simulink model "car_model_spl_heur3"  (R2020b)
settings: Solver=FixedStepAuto  StartTime=0.0  StopTime=45  FixedStep=0.05  RelTol=1e-3
undefined symbols (not defined in the file or in its folder): theta0, x0, y0
settings Model: Creator=Lexa  LastModifiedBy=msw
settings SolverCC: AlgebraicLoopSolver=LineSearch
settings DebuggingCC: UnderSpecifiedDimensionMsg=error
settings SFSimCC: CustomCodeUndefinedFunction=UseInterfaceOnly

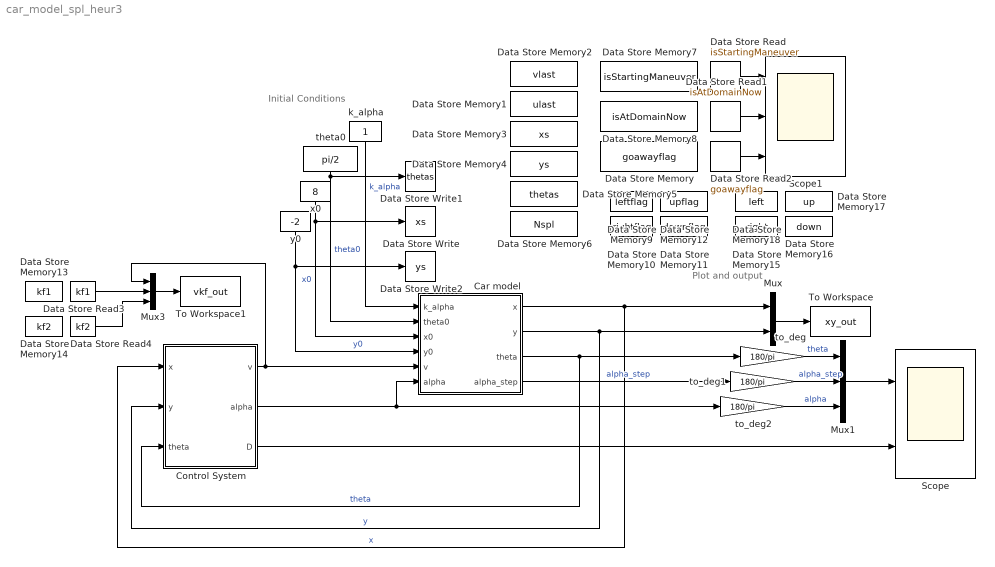
== system car_model_spl_heur3 ==
  note: Plot and output
  note: Initial Conditions
  Car model : Subsystem
      mask Display: image('car_model.png');
  Control System : Subsystem  StopFcn=close all
  Data Store Memory : DataStoreMemory  DataStoreName=goawayflag  ReadBeforeWriteMsg=warning  WriteAfterWriteMsg=warning  WriteAfterReadMsg=warning  ShowAdditionalParam=off  OutDataTypeStr=double
  Data Store Memory1 : DataStoreMemory  DataStoreName=ulast  ReadBeforeWriteMsg=warning  WriteAfterWriteMsg=warning  WriteAfterReadMsg=warning  ShowAdditionalParam=off  OutDataTypeStr=double
  Data Store Memory10 : DataStoreMemory  DataStoreName=rightflag  ReadBeforeWriteMsg=warning  WriteAfterWriteMsg=warning  WriteAfterReadMsg=warning  ShowAdditionalParam=off  OutDataTypeStr=double
  Data Store Memory11 : DataStoreMemory  DataStoreName=downflag  ReadBeforeWriteMsg=warning  WriteAfterWriteMsg=warning  WriteAfterReadMsg=warning  ShowAdditionalParam=off  OutDataTypeStr=double
  Data Store Memory12 : DataStoreMemory  DataStoreName=upflag  ReadBeforeWriteMsg=warning  WriteAfterWriteMsg=warning  WriteAfterReadMsg=warning  ShowAdditionalParam=off  OutDataTypeStr=double
  Data Store Memory13 : DataStoreMemory  DataStoreName=kf1  ReadBeforeWriteMsg=warning  WriteAfterWriteMsg=warning  WriteAfterReadMsg=warning  ShowAdditionalParam=off  OutDataTypeStr=double
  Data Store Memory14 : DataStoreMemory  DataStoreName=kf2  ReadBeforeWriteMsg=warning  WriteAfterWriteMsg=warning  WriteAfterReadMsg=warning  ShowAdditionalParam=off  OutDataTypeStr=double
  Data Store Memory15 : DataStoreMemory  DataStoreName=right  ReadBeforeWriteMsg=warning  WriteAfterWriteMsg=warning  WriteAfterReadMsg=warning  ShowAdditionalParam=off  OutDataTypeStr=double
  Data Store Memory16 : DataStoreMemory  DataStoreName=down  ReadBeforeWriteMsg=warning  WriteAfterWriteMsg=warning  WriteAfterReadMsg=warning  ShowAdditionalParam=off  OutDataTypeStr=double
  Data Store Memory17 : DataStoreMemory  DataStoreName=up  ReadBeforeWriteMsg=warning  WriteAfterWriteMsg=warning  WriteAfterReadMsg=warning  ShowAdditionalParam=off  OutDataTypeStr=double
  Data Store Memory18 : DataStoreMemory  DataStoreName=left  ReadBeforeWriteMsg=warning  WriteAfterWriteMsg=warning  WriteAfterReadMsg=warning  ShowAdditionalParam=off  OutDataTypeStr=double
  Data Store Memory2 : DataStoreMemory  DataStoreName=vlast  ReadBeforeWriteMsg=warning  WriteAfterWriteMsg=warning  WriteAfterReadMsg=warning  ShowAdditionalParam=off  OutDataTypeStr=double
  Data Store Memory3 : DataStoreMemory  DataStoreName=xs  ReadBeforeWriteMsg=warning  WriteAfterWriteMsg=warning  WriteAfterReadMsg=warning  ShowAdditionalParam=off  OutDataTypeStr=double
  Data Store Memory4 : DataStoreMemory  DataStoreName=ys  ReadBeforeWriteMsg=warning  WriteAfterWriteMsg=warning  WriteAfterReadMsg=warning  ShowAdditionalParam=off  OutDataTypeStr=double
  Data Store Memory5 : DataStoreMemory  DataStoreName=thetas  ReadBeforeWriteMsg=warning  WriteAfterWriteMsg=warning  WriteAfterReadMsg=warning  ShowAdditionalParam=off  OutDataTypeStr=double
  Data Store Memory6 : DataStoreMemory  DataStoreName=Nspl  ReadBeforeWriteMsg=warning  WriteAfterWriteMsg=warning  WriteAfterReadMsg=warning  ShowAdditionalParam=off  OutDataTypeStr=double
  Data Store Memory7 : DataStoreMemory  DataStoreName=isStartingManeuver  ReadBeforeWriteMsg=warning  WriteAfterWriteMsg=warning  WriteAfterReadMsg=warning  ShowAdditionalParam=off  OutDataTypeStr=double
  Data Store Memory8 : DataStoreMemory  DataStoreName=isAtDomainNow  ReadBeforeWriteMsg=warning  WriteAfterWriteMsg=warning  WriteAfterReadMsg=warning  ShowAdditionalParam=off  OutDataTypeStr=boolean
  Data Store Memory9 : DataStoreMemory  DataStoreName=leftflag  ReadBeforeWriteMsg=warning  WriteAfterWriteMsg=warning  WriteAfterReadMsg=warning  ShowAdditionalParam=off  OutDataTypeStr=double
  Data Store Read : DataStoreRead  DataStoreName=isStartingManeuver
  Data Store Read1 : DataStoreRead  DataStoreName=isAtDomainNow
  Data Store Read2 : DataStoreRead  DataStoreName=goawayflag
  Data Store Read3 : DataStoreRead  DataStoreName=kf1
  Data Store Read4 : DataStoreRead  DataStoreName=kf2
  Data Store Write : DataStoreWrite  DataStoreName=xs
  Data Store Write1 : DataStoreWrite  DataStoreName=thetas
  Data Store Write2 : DataStoreWrite  DataStoreName=ys
  Mux : Mux  Inputs=2
  Mux1 : Mux  Inputs=3
  Mux3 : Mux  Inputs=3
  Scope : Scope  NumInputPorts=2
  Scope1 : Scope  NumInputPorts=3
  To Workspace : ToWorkspace  VariableName=xy_out  SaveFormat=Timeseries  SampleTime=-1
  To Workspace1 : ToWorkspace  VariableName=vkf_out  SaveFormat=Timeseries  SampleTime=-1
  k_alpha : Constant  VectorParams1D=off
  theta0 : Constant  Value=pi/2  VectorParams1D=off
  to_deg : Gain  Gain=180/pi
  to_deg1 : Gain  Gain=180/pi
  to_deg2 : Gain  Gain=180/pi
  x0 : Constant  Value=8
  y0 : Constant  Value=-2
  wires:
  Mux/1 -> To Workspace/1
  Car model/1(x) -> Control System/1(x), Mux/1  "x"
  Car model/2(y) -> Control System/2(y), Mux/2  "y"
  theta0/1 -> Data Store Write1/1, Car model/2(theta0)  "theta0"
  x0/1 -> Data Store Write/1, Car model/3(x0)  "x0"
  y0/1 -> Data Store Write2/1, Car model/4(y0)  "y0"
  to_deg/1 -> Mux1/1  "theta"
  Car model/4(alpha_step) -> to_deg1/1  "alpha_step"
  to_deg1/1 -> Mux1/2  "alpha_step"
  to_deg2/1 -> Mux1/3  "alpha"
  Mux1/1 -> Scope/1
  Car model/3(theta) -> Control System/3(theta), to_deg/1  "theta"
  Control System/2(alpha) -> Car model/6(alpha), to_deg2/1
  Control System/3(D) -> Scope/2
  Control System/1(v) -> Car model/5(v), Mux3/1
  Data Store Read/1 -> Scope1/1
  Data Store Read1/1 -> Scope1/2
  Data Store Read2/1 -> Scope1/3
  Data Store Read3/1 -> Mux3/2
  Mux3/1 -> To Workspace1/1
  Data Store Read4/1 -> Mux3/3
  k_alpha/1 -> Car model/1(k_alpha)  "k_alpha"

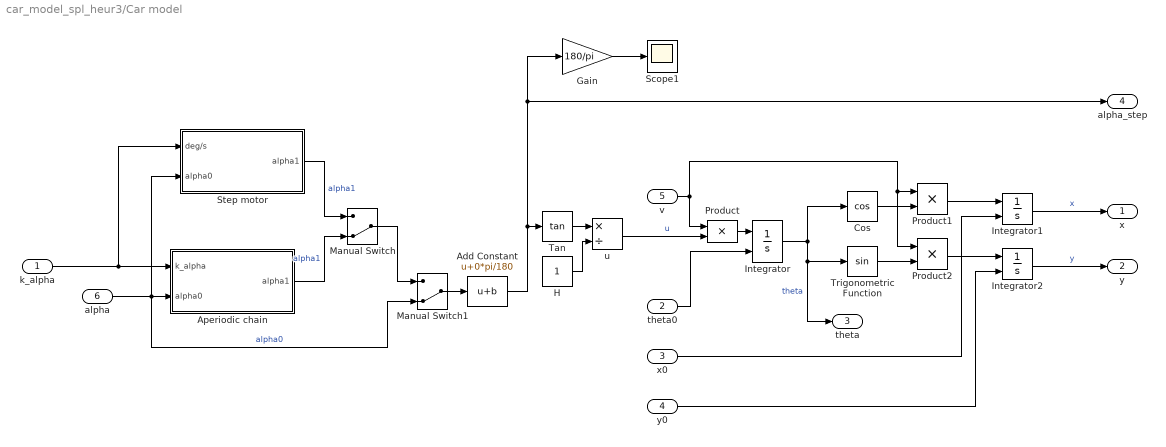
== system car_model_spl_heur3/Car model ==
  k_alpha : Inport
  theta0 : Inport  Port=2
  x0 : Inport  Port=3
  y0 : Inport  Port=4
  v : Inport  Port=5
  alpha : Inport  Port=6
  Add Constant : Bias  Bias=0*pi/180
  Aperiodic chain : Subsystem
  Cos : Trigonometry  Operator=cos
  Gain : Gain  Gain=180/pi
  H : Constant  VectorParams1D=off
  Integrator : Integrator  InitialConditionSource=external  InitialCondition=theta0  WrapState=on
  Integrator1 : Integrator  InitialConditionSource=external  InitialCondition=x0
  Integrator2 : Integrator  InitialConditionSource=external  InitialCondition=y0
  Manual Switch : ManualSwitch  CurrentSetting=0
  Manual Switch1 : ManualSwitch  CurrentSetting=0
  Product : Product
  Product1 : Product
  Product2 : Product
  Scope1 : Scope
  Step motor : Subsystem
  Tan : Trigonometry  Operator=tan
  Trigonometric Function : Trigonometry
  u : Product  Inputs=*/
  x : Outport  VectorParamsAs1DForOutWhenUnconnected=off
  y : Outport  Port=2  VectorParamsAs1DForOutWhenUnconnected=off
  theta : Outport  Port=3  VectorParamsAs1DForOutWhenUnconnected=off
  alpha_step : Outport  Port=4  VectorParamsAs1DForOutWhenUnconnected=off
  wires:
  x0/1 -> Integrator1/2
  Product/1 -> Integrator/1
  Trigonometric Function/1 -> Product2/2
  v/1 -> Product2/1, Product1/1, Product/1
  Integrator/1 -> theta/1, Trigonometric Function/1, Cos/1  "theta"
  Integrator2/1 -> y/1  "y"
  y0/1 -> Integrator2/2
  Integrator1/1 -> x/1  "x"
  Cos/1 -> Product1/2
  Product1/1 -> Integrator1/1
  Product2/1 -> Integrator2/1
  theta0/1 -> Integrator/2
  H/1 -> u/2
  Tan/1 -> u/1
  u/1 -> Product/2  "u"
  alpha/1 -> Manual Switch1/2, Aperiodic chain/2(alpha0), Step motor/2(alpha0)  "alpha0"
  Manual Switch1/1 -> Add Constant/1
  Gain/1 -> Scope1/1
  k_alpha/1 -> Aperiodic chain/1(k_alpha), Step motor/1(deg/s)
  Step motor/1(alpha1) -> Manual Switch/1  "alpha1"
  Aperiodic chain/1(alpha1) -> Manual Switch/2  "alpha1"
  Manual Switch/1 -> Manual Switch1/1
  Add Constant/1 -> Gain/1, alpha_step/1, Tan/1

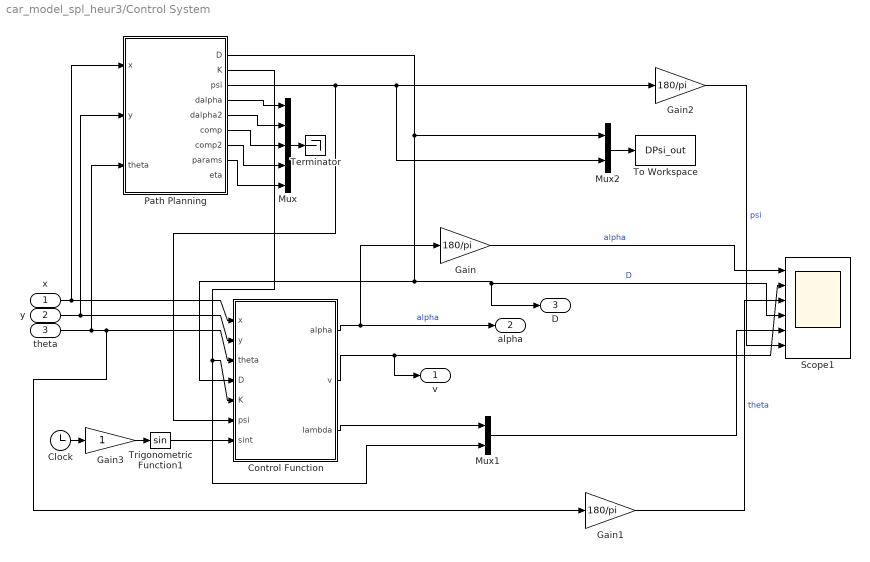
== system car_model_spl_heur3/Control System ==
  x : Inport
  y : Inport  Port=2
  theta : Inport  Port=3
  Clock : Clock
  Control Function : MATLAB Function  TreatAsAtomicUnit=on
  Gain : Gain  Gain=180/pi
  Gain1 : Gain  Gain=180/pi
  Gain2 : Gain  Gain=180/pi
  Gain3 : Gain
  Mux : Mux  Inputs=5
  Mux1 : Mux  Inputs=2
  Mux2 : Mux  Inputs=2
  Path Planning : MATLAB Function  TreatAsAtomicUnit=on
  Scope1 : Scope  NumInputPorts=6
  Terminator : Terminator
  To Workspace : ToWorkspace  VariableName=DPsi_out  SaveFormat=Timeseries  SampleTime=-1
  Trigonometric Function1 : Trigonometry
  v : Outport  VectorParamsAs1DForOutWhenUnconnected=off
  alpha : Outport  Port=2  VectorParamsAs1DForOutWhenUnconnected=off
  D : Outport  Port=3  VectorParamsAs1DForOutWhenUnconnected=off
  wires:
  theta/1 -> Gain1/1, Control Function/3(theta), Path Planning/3(theta)
  Path Planning/1(D) -> Control Function/4(D), Scope1/4, D/1, Mux2/1  "D"
  Control Function/1(alpha) -> alpha/1, Gain/1  "alpha"
  y/1 -> Control Function/2(y), Path Planning/2(y)
  x/1 -> Path Planning/1(x), Control Function/1(x)
  Gain/1 -> Scope1/1  "alpha"
  Path Planning/2(K) -> Mux1/2, Control Function/5(K)
  Path Planning/4(dalpha) -> Mux/1
  Path Planning/5(dalpha2) -> Mux/2
  Path Planning/6(comp) -> Mux/3
  Path Planning/7(comp2) -> Mux/4
  Path Planning/8(params) -> Mux/5
  Gain1/1 -> Scope1/3  "theta"
  Gain2/1 -> Scope1/6  "psi"
  Control Function/3(lambda) -> Mux1/1
  Mux1/1 -> Scope1/5
  Mux2/1 -> To Workspace/1
  Control Function/2(v) -> v/1, Scope1/2
  Mux/1 -> Terminator/1
  Path Planning/3(psi) -> Gain2/1, Mux2/2, Control Function/6(psi)
  Clock/1 -> Gain3/1
  Gain3/1 -> Trigonometric Function1/1
  Trigonometric Function1/1 -> Control Function/7(sint)

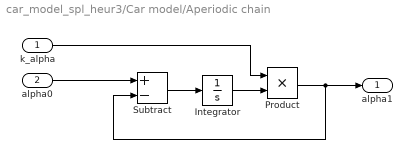
== system car_model_spl_heur3/Car model/Aperiodic chain ==
  k_alpha : Inport
  alpha0 : Inport  Port=2
  Integrator : Integrator
  Product : Product
  Subtract : Sum  Inputs=+-
  alpha1 : Outport  VectorParamsAs1DForOutWhenUnconnected=off
  wires:
  alpha0/1 -> Subtract/1
  Subtract/1 -> Integrator/1
  Integrator/1 -> Product/2
  Product/1 -> Subtract/2, alpha1/1
  k_alpha/1 -> Product/1

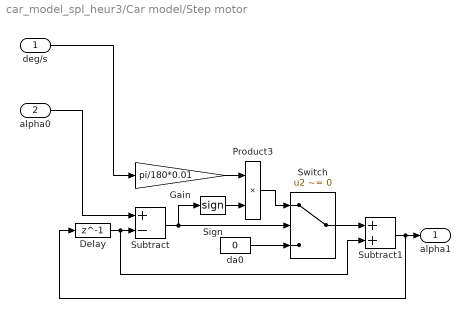
== system car_model_spl_heur3/Car model/Step motor ==
  deg/s : Inport
  alpha0 : Inport  Port=2
  Delay : Delay  DelayLength=1  InitialCondition=0
  Gain : Gain  Gain=pi/180*0.01
  Product3 : Product
  Sign : Signum
  Subtract : Sum  Inputs=+-
  Subtract1 : Sum
  Switch : Switch  Criteria=u2 ~= 0
  da0 : Constant  Value=0  VectorParams1D=off
  alpha1 : Outport  VectorParamsAs1DForOutWhenUnconnected=off
  wires:
  Delay/1 -> Subtract1/2, Subtract/2
  da0/1 -> Switch/3
  deg/s/1 -> Gain/1
  Product3/1 -> Switch/1
  alpha0/1 -> Subtract/1
  Sign/1 -> Product3/2
  Subtract/1 -> Sign/1, Switch/2
  Switch/1 -> Subtract1/1
  Subtract1/1 -> Delay/1, alpha1/1
  Gain/1 -> Product3/1

== matlab function car_model_spl_heur3/Control System/Control Function ==
  settings: updateMethod=DISCRETE
  data: x input; alpha output; y input; theta input size=1; D input; K input; psi input; sint input size=1; vlast data_store_memory; ulast data_store_memory; goawayflag data_store_memory; xs data_store_memory; ys data_store_memory; thetas data_store_memory; v output; isStartingManeuver data_store_memory; isAtDomainNow data_store_memory; leftflag data_store_memory; rightflag data_store_memory; upflag data_store_memory; downflag data_store_memory; lambda output; kf1 data_store_memory; kf2 data_store_memory; left data_store_memory; right data_store_memory; up data_store_memory; down data_store_memory
function [alpha, v, lambda] = fcn(x,y,theta, D, K, psi, sint)

global goawayflag;
global leftflag;
global rightflag;
global upflag;
global downflag;
global left;
global right;
global up;
global down;
global isStartingManeuver;
global isAtDomainNow;
global ulast;
global vlast;
global xs;
global ys;
global thetas;
global Nspl;
global kf1;
global kf2;

lambda = 2;
H = 0.75; % between front and back
% thrhld = 20*pi/180;
% Rmin = H/tan(thrhld);
Rmin = 2;
thrhld = atan(H/Rmin);

isAtDomainNow = isAtDomain(D, psi);

% Rgoaway = 2.5*Rmin;

%% leftrightflags
if(vlast == 0)
%     left = 0.5;
%     up = 0.5*Rmin;
%     right = max(xs+0.5*Rmin, left+1*Rmin);
%     down = min(ys-0.25*Rmin, up-1.5*Rmin);
    up = -0.2;
    right = 8+1*Rmin;
    left = min(xs-0.25*Rmin, right-1.25*Rmin);
    down = min(ys-0.5*Rmin, up-1*Rmin);
end

% if(x+1*Rmin < right)
%     right = max(x+1*Rmin, right-1*Rmin);
% end
if(y-0.25*Rmin > down)
    down = min(y-0.25*Rmin, up-1.1*Rmin);
end
if(x-0.25*Rmin > left)
    left = min(x-0.25*Rmin, right-2*Rmin);
end


if (x < left)
    leftflag = 1;
    rightflag = 0;
end

if (x > right)
    leftflag = 0;
    rightflag = 1;
end

if (y > up)
    upflag = 1;
    downflag = 0;
end

if (y < down)
    upflag = 0;
    downflag = 1;
end

% subplot(2,1,1)
line([left, right], [down, down], 'Color','red','LineStyle','--'); 
line([left, right], [up, up], 'Color','red','LineStyle','--');
line([left, left], [down, up], 'Color','red','LineStyle','--');
line([right, right], [down, up], 'Color','red','LineStyle','--');
% plot(r_obs(1), r_obs(2), 'ko')

%% heuristics
P0 = [59.332830061664560,34.913367956132944;34.913367956132944,36.199614068700980];
% P0 = [2.71604432159105,1.48162473482028;1.48162473482028,2.37197445604761];

if (isStartingManeuver) && (~isAtDomainNow)
    if(vlast == 0)
        v = + 0.5;
        
%     kf1 =  + 2*0.5 / 0.5^2 ;
%     kf2 =  - 2*0.5 / 0.5^2 ;
        
%     kf1 =  + 2*0.5 / 0.5^2;
%     kf2 =  + 2*0.5 / 0.5^2 + 50;
%     kf2 =  + 2*0.5 / 0.5^2 - 30;
%     kf2 = -kf1;

%     kf1 = 1/(tan(thetas)/ys+0.08);
%     kf2 = 1/(tan(thetas)/ys-0.08);

    else
        v = vlast;
    end
   
        
    if(leftflag)
        v = - vlast; 
        leftflag = 0;
    end

    if(rightflag)
        v = - vlast;
        rightflag = 0;
    end

    if(downflag)
        v = - vlast; 
        downflag = 0;
    end

    if(upflag)
        v = - vlast;
        upflag = 0;
    end

    

%% C.Samson

%     if (abs(psi) < pi/3)
% %         k1 = 0*1.2;
%         k2 = 10;
%         k3 = 18;
%         alph = 3;
% 
% %         z1 = x;
%         z2 = D;
%         z3 = tan(psi);
%         % kfsin = alph*norm([z2,z3]);
%         % kfsin = norm([z2,z3]);
%         kfsin = 1;
% 
%         v = (+kfsin*sint)/cos(psi);
%         u = (cos(psi))^3*(-k2*z2 - sign(v*cos(psi))*k3*z3);
% 
%         alpha = atan2(u*H,1);
%     else
%         if (v >= 0)
%             alpha = -psi;
%         else
%             alpha = +psi;
%         end
%     end

%% Feedback linearization starting maneuver
    lambda_loc = 2;
    sigma_loc1 = 2*lambda_loc*sin(psi)+lambda_loc*lambda_loc*D;
    
%     if (abs(psi) < pi/2)
%         if (v >= 0)
%             if (abs(D) < Rmin)
%                 u = (-sigma_loc1)/cos(psi);
%                 alpha = atan2(u*H,1);
%             else
%                 alpha = -psi+pi/2*sign(psi);
%             end
%         else
% %             u = 0;
% %             alpha = atan2(u*H,1);            
%             if (abs(D) < Rmin)
%                 alpha = +psi;
%             else
%                 alpha = -psi;
%             end
%         end
%     else
%         if (v >= 0)
%             alpha = -psi;
%         else
%             alpha = +psi;
%         end
%     end

if sign(thetas)~=0
    sigths = sign(thetas);
else
    sigths = 1;
end
u = 0;
% if (abs(D) < Rmin/2)
if (abs(D) < 2*Rmin/3)
    if (v >= 0)
        if (abs(psi) < pi/2)
            u = (-sigma_loc1)/cos(psi);
            alpha = atan2(u*H,1);
        else
            alpha = -psi;
        end
    else
        alpha = +psi;
    end
else
    if (v >= 0)
%             alpha = -sign(abs(psi)-pi/2)*abs(abs(psi)-pi/2)^2;
        alpha = sigths*(abs(psi)-pi/2);
    else
%             alpha = sign(abs(psi)-pi/2)*abs(abs(psi)-pi/2)^2;
        alpha = -sigths*(abs(psi)-pi/2);
    end
end
    
elseif (1)
%% continue with spline following
    %% Spline
    sigma = 2*lambda*sin(psi)+lambda*lambda*D;
    v = 0.6;
    
%     u = K*cos(psi)/(K*D+1) + (-sigma)/cos(psi);
%     alpha = atan2(u*H,1);
    
    ro = [8.0; 4.0];
    hold on
    plot(ro(1), ro(2), 'ko')
    hold off
    
    rmin = 2;
    mu = 0.5;
    ev = [cos(theta); sin(theta)];
    evx = [-sin(theta) cos(theta)];
    r = [x; y];
    dr = ro - r;
    drs = -ev;
    ndr = norm(dr);
    ndrs = -ev' * dr / ndr; % checkon 0
    
    cosTheta = dot(ev, dr/ndr);
    sinThetaSq = 1 - cosTheta^2;
    if ndr > rmin
        Pi = 0;
        Pis = 0;
        Piss = 0;
        u = u_obs_pot_generated2_off(K,mu,psi,D,sin(psi));
    else
        Pi = 0.5*(rmin - ndr)^2;
        Pis = -(rmin - ndr)*ndrs;
        Piss = 0;
        hold on
        plot(ro(1), ro(2), 'r*')
        hold off
%         Pimult, ev1,ev2,evx1,evx2,k,mu,ndr,psi,r1,r2,rmin,ro1,ro2,z1,z2
        Pi_mult = 10;
%         u = u_obs_pot_generated2(Pi_mult, ev(1),ev(2),evx(1),evx(2),K,mu,ndr,psi,r(1),r(2),rmin,ro(1),ro(2),sinThetaSq,D,sin(psi));
        u = u_template2(Pi_mult, ro, K, D, psi, r, theta, rmin);
    end
%     u = u_obs_pot_generated2_off(K,mu,psi,D,sin(psi));
else
    error('NotAttrDomain');
end

alpha = atan2(u*H,1);
if isnan(alpha)
    alpha = 0;
end
thrhld = 20 * pi / 180;
if alpha>=thrhld
    alpha=thrhld;
elseif alpha<-thrhld
    alpha=-thrhld;
end     
u = tan(alpha)/H;

ulast = u;
vlast = v;

%% Auxilairy functions

function isAttrDomain = isAtDomain(D, psi)
%% Attraction Domain
z1 = D;
z2 = tan(psi);
%% old (big) domain
% P = [0.145601915600065,0.172247944870462;0.172247944870462,0.516852979587000];
% 
% isAttrDomain = (z'*P*z <=1) && (abs(psi)<pi/2);
%% single domain
lambda = 2; %mu = 0.6*lambda
theta2 = 0;
P = [61.6719821815400,31.8444380141815;31.8444380141815,26.2774420451554];
P = [1.924902434656336e+02,89.167566356124900;89.167566356124900,86.056817553176230];
Rmin = 1/0.5;

% [168.581046629451,86.8576492929144;86.8576492929144,110.004902211710]

isAttrDomain = (Vfun(z1, z2, theta2, 1/Rmin, [lambda*lambda; 2*lambda], P) <= 100) && (abs(psi)<pi/2);
%% triple domain
% P08 = [36.015276255922110,27.294581971649464;27.294581971649464,67.657754995904200]; %alpha1 = 0.2
% lambda08 = 0.8; theta08 = -44.228974888947740;
% 
% P1 = [39.815052334731924,30.021201049505690;30.021201049505690,60.930005254749450]; %alpha1 = 0.2
% lambda1 = 1; theta1 = -26.727990955940450;
% 
% P15 = [53.590138212703700,38.794377319214800;38.794377319214800,53.207560182062420]; %alpha1 = 0.2
% lambda15 = 1.5; theta15 = -10.986753437494730;
% 
% P2 = [59.332830061664560,34.913367956132944;34.913367956132944,36.199614068700980]; %alpha1 = 0.2
% lambda2 = 2; theta2 = -4.231907625174246;
% 
% 
% if (Vfun(z1, z2, theta08, 1/Rmin, [lambda08^2; 2*lambda08], P08) <= 1)
%     lambda = 0.8; 
%     attr = 1;
% elseif (Vfun(z1, z2, theta1, 1/Rmin, [lambda1^2; 2*lambda1], P1) <= 1)
%     lambda = 1; 
%     attr = 1;
% elseif (Vfun(z1, z2, theta15, 1/Rmin, [lambda15^2; 2*lambda15], P15) <= 1)
%     lambda = 1.5;
%     attr = 1;
% elseif (Vfun(z1, z2, theta2, 1/Rmin, [lambda2^2; 2*lambda2], P2) <= 1)
%     lambda = 2; 
%     attr = 1;
% else
%     attr = 0;
% end
% isAttrDomain = (attr) && (abs(psi)<pi/2);
end


function val = Vfun(z1, z2, theta, umax, c, P)
    z = [z1 ;z2 ];
    sigma = c'*z;
    if sigma >= umax*(1+z2 *z2 )^1.5   
        addval = theta*(umax*(1+z2 *z2 )^1.5)*(sigma-0.5*umax*(1+z2 *z2 )^1.5);
    elseif sigma <= -umax*(1+z2 *z2 )^1.5   
        addval = theta*(umax*(1+z2 *z2 )^1.5)*(-sigma-0.5*umax*(1+z2 *z2 )^1.5);
    else %if abs(sigma) < umax*(1+z2*z2)^1.5
        addval = theta*(sigma^2)/2;
    end

    val = z'*P*z + addval;
end

end

== matlab function car_model_spl_heur3/Control System/Path Planning ==
  settings: updateMethod=DISCRETE
  data: D output size=1; K output; x input; psi output; y input; theta input size=1; vlast data_store_memory; ulast data_store_memory; goawayflag data_store_memory; xs data_store_memory; ys data_store_memory; thetas data_store_memory; Nspl data_store_memory; isStartingManeuver data_store_memory; dalpha output; dalpha2 output; comp output; comp2 output; params output; isAtDomainNow data_store_memory; eta output
function [D,K,psi, dalpha, dalpha2, comp, comp2, params,eta] = fcn(x,y,theta)
eta = 0;
% if(isempty(Snum))
%     Snum = 0;
% end

%% CONSTANTS

global goawayflag;
global isStartingManeuver;
global isAtDomainNow;
global xs;
global ys;
global thetas;
global Nspl;
global vlast;


H = 0.7; % between front and back
thrhld = 30*pi/180;
Rmin = H/tan(thrhld);

Rgoaway = 2.5*Rmin;

%% DESIRED TRAJECTORY

% input0 = [0,0;-37.7033999999985,-11.6936999997124;-46.6699999999255,-13.1520999995992;-48.4167728694156,-14.4249271200970;-49.7144662700594,-15.2920181304216;-51.2451999997720,-15.5964999999851;-52.7759337294847,-15.2920181304216;-54.0736271198839,-14.4249271200970;-54.9407181302086,-13.1272337296978;-55.2451999997720,-11.5964999999851;-54.9407181302086,-10.0657662702724;-54.0736271198839,-8.76807286962867;-52.7759337294847,-7.90098186954856;-51.2451999997720,-7.59649999998510;-49.7144662700594,-7.90098186954856;-48.4167728694156,-8.76807286962867;-45.8026000000536,-11.0564000001177;-41.2840999998152,-11.4974999995902;-36.3594999993220,-10.7231000000611;-1.24519999977201,0.230100000277162];
% input0 = [0,0;-1,0;-2,-0.25;-3,0;-4,0.2;-5,0.5;-6,0.3];
input0 = [8.21600326006528,0;8.21600326006528,2.98925005022913;8.20758457882733,5.98628231571288;8.69140109578713,8.06028145277067;10.1710371562285,9.59202163069941;12.2270574729172,10.1472975092063;14.2766380038332,9.56870396277120;15.7387802050626,8.02025602141151;16.1990078075244,5.94089520714774;15.5268592055012,3.92006193799355;13.9128696601541,2.53060571605069;11.5072489414890,1.05548560520278];

inputPs = input0(1,:);
inputPe = input0(end,:);
input = [2*inputPs-input0(2,:); input0; 2*inputPe-input0(end-1,:)];

M = 1/6*[1, -3, 3, -1;
         4, 0, -6, 3;
         1, 3, 3, -3;
         0, 0, 0, 1];
     
     
input2 = [];     
for Nspl2 = 2 :1: (size(input,1)-2) 
    for t=0:0.1:1
        input2 =  [input2, r(Nspl2,t)];
    end
end     
input2 = input2';     

%% PATH PLANNING
X = [x;y];
Xs = [xs;ys];
orient = [cos(theta);sin(theta)];
%% target start of trajectory
Pspl = r(2,0);
dPspl = dr(2,0);
x0 = Pspl(1);
y0 = Pspl(2);
tau0 = AngSign([1;0], dPspl); 

%% GoAwayFlag
if (x == xs) && (y == ys)
%     subplot(2,1,2); hold off;    
end

if ((xs-x0)^2+(ys-y0)^2 <= (Rgoaway)^2) && (x == xs) && (y == ys)
    goawayflag = 1;
end

if ((x-x0)^2+(y-y0)^2 > (Rgoaway)^2)
    goawayflag = 0;
end

%% CALCULATION DKPsi
if ((Xs - Pspl)'*dPspl < 0)
    isStartingManeuver = 1;
end

if ((X - Pspl)'*dPspl < 0) % We are moving behind of spline starting point - construct the line and follow it.
    D = distPLsign(X, Pspl, dPspl);
    K = 0;
    psi = AngSign(dPspl,orient);
    
    %% PLOT
%     subplot(2,1,1)
    plot(input0(:,1),input0(:,2), 'square'); daspect([1 1 1]); grid on; hold on;
    plot(input2(:,1),input2(:,2), 'b-');
else % We are moving on the spline
    D = 0;
    K = 0;
    psi = 0;
    
    phi = 0; PHI = 0; Xc = [inf; inf]; XL = [0; 0]; Xcplot = [0;0]; Xtauplot = [0;0]; %% ---->>> WTF? %%
    isStartingManeuver = 0;
    
    while( Nspl<=(size(input,1)-2))
        if Nspl < 2
            Nspl = 2;
        end
        
        Xc = NorCrossPnt(r(Nspl,0),dr(Nspl,0),r(Nspl,1),dr(Nspl,1));

        if ( (isinf(Xc(1)) || isinf(Xc(2))) )  % ----->>>>> !! -> THIS IS MISTAKE -> !!norm(r(Nspl,0)-Xc) > 500 % K(0) < 1/200
            PHI = norm(r(Nspl,1)-r(Nspl,0));
            XL = CrossPnt(X,NormVec(dr(Nspl,0)),r(Nspl,0),dr(Nspl,0));
            phi = norm(XL-r(Nspl,0)); %*cos(AngbwVec(XL-r(Nspl,0),r(Nspl,0)));
            Xcplot = XL+NormVec(dr(Nspl,0))/norm(NormVec(dr(Nspl,0)));
            Xtauplot = XL+dr(Nspl,0)/norm(dr(Nspl,0));
            Xc = [inf; inf];
        else
            PHI = AngSign(r(Nspl,0)-Xc, r(Nspl,1)-Xc)*180/pi; 
            phi = AngSign(r(Nspl,0)-Xc, X-Xc)*180/pi; 
            phi = phi*sign(PHI);
            PHI = PHI*sign(PHI);
        end

        if phi>PHI
            Nspl = Nspl+1;
        elseif phi<= PHI && phi>=0
            break;
        elseif phi<0
%             error('phi<0');
            Nspl = Nspl-1;
        end
    end

    if Nspl < 2
        error('Behind of spline start');
    elseif Nspl > (size(input,1)-2) 
        error('End of spline'); 
    else
        [eta, D,K,psi] = DKPsi(X,orient, @(t)calcEta(Nspl,t), @(t)r(Nspl,t),@(t)dr(Nspl,t),@(t)ddr(Nspl,t),phi,PHI,Xc);
    end
    %% PLOT
    step = 0.05;
    plot(input0(:,1),input0(:,2), 'square'); daspect([1 1 1]); grid on; hold on;
    plot(input2(:,1),input2(:,2), 'b-');
    
    output = [];
    for t=0:step:1
        output =  [output, r(Nspl,t)];
    end
    output = output';
    plot(output(:,1),output(:,2),'LineWidth', 3); daspect([1 1 1]); grid on; hold on; ylim([min(input0(:,2))-1; max(input0(:,2))+1]); xlim([min(input0(:,1))-1; max(input0(:,1))+1]);

    plot(X(1),X(2),'ok', 'MarkerSize', 10, 'MarkerFaceColor', 'g');
    if(~((isinf(Xc(1)) || isinf(Xc(2)))))
    plot(Xc(1),Xc(2), 'rx');
    PlotLine(r(Nspl,0),Xc);
    PlotLine(r(Nspl,1),Xc);
    PlotLine(X,Xc);
    else
    plot(XL(1),XL(2), 'o');
    plot(Xcplot(1),Xcplot(2), 'b^');
    plot(Xtauplot(1),Xtauplot(2), 'm<');
    end
    hold off;

end

%% Starting Maneuver
if (isStartingManeuver)
    
    if AngSign(dPspl, Xs-Pspl) < 0
        params = +1;
%     elseif (AngSign(dPspl, Xs-Pspl) == pi) % -----<<< IS THIS MISTAKE  ANGSIGN? >>>-----
%         params = 0;
    else %if AngSign(dPspl, Xs-Pspl) > 0 
        params = -1;
    end

    if AngSign(dPspl, X-Pspl) < 0
        param = +1;
%     elseif (AngSign(dPspl, X-Pspl) == pi)  %v-----<<< IS THIS MISTAKE  ANGSIGN? >>>-----
%         param = 0;
    else %if AngSign(dPspl, X-Pspl) > 0
        param = -1;
    end


    %  target circle radius and tangent vector
    if (AngSign(dPspl, Xs-Pspl) == 0)
        tangent = dPspl;
        R = inf;
    else
        [X0,Y0,R] = BuildCircle(x,y,x0,y0,tau0); %% ----->>>>---- подредактировать внутри на предмет предельных значений -----<<<<<----

        dx = X0 - x; 
        dy = Y0 - y;

        if (R < Rmin) 
            tangent = dPspl;
        else   
            tangent = NormVec([dx;dy], param)/norm(NormVec([dx;dy], param));


%         dphi = 0:pi/180:2*pi;
%         xplot = R*cos(dphi) + X0; 
%         yplot = R*sin(dphi) + Y0;
%         plot(xplot, yplot); hold on;


        end
    end

    dalpha = AngSign(tangent,[cos(theta);sin(theta)]);
%     dalpha2 = AngSign([x0;y0] - 2*Rgoaway*[cos(tau0+params*pi/2.5);sin(tau0+params*pi/2.5)],[cos(theta);sin(theta)]);
    dalpha2 = pi + psi - params*pi/2.5;
    comp = tangent'*orient;
    comp2 = dPspl'*orient;
    
    comp = x;
    comp2 = y;
    dalpha = theta;
    %% PLOTS
%     subplot(2,1,1)
%     Radii = NormVec(dPspl,-params)/norm(NormVec(dPspl,-params));
%     X0 = x0 + Rmin*Radii(1);
%     Y0 = y0 + Rmin*Radii(2);
% 
%     dphi = 0:pi/18:2*pi;
%     xplot = Rmin*cos(dphi) + X0; 
%     yplot = Rmin*sin(dphi) + Y0;
% 
%     plot(xplot, yplot); hold on; grid on; daspect([1 1 1]);
%     plot(X0,Y0,'x');
    line([x0, x0+cos(tau0)], [y0, y0+sin(tau0)], 'Color','red','LineStyle','-'); hold on;

%     xplot = Rgoaway*cos(dphi) + x0; 
%     yplot = Rgoaway*sin(dphi) + y0;
%     plot(xplot, yplot);

    line([x, x+cos(theta)], [y, y+sin(theta)], 'Color','black','LineStyle','--');
 
    if(isAtDomainNow)
        plot(x,y,'ok', 'MarkerSize', 10, 'MarkerFaceColor', 'g');
        sprintf("continue with spline, z1 = %.3f; z2 = %.3f; psi = %.1f;", D, tan(psi), psi*180/pi);
    elseif ( vlast<0 )
        plot(x,y,'ok', 'MarkerSize', 10, 'MarkerFaceColor', 'r');
    else
        plot(x,y,'ok', 'MarkerSize', 10, 'MarkerFaceColor', 'y');
    end

    xlim([x-5;x+5]);
    ylim([y-5;y+5]);
    hold off;

%     subplot(2,1,2)
%     grid on;
%     if ( vlast<0 )
%         plot(D,tan(psi),'.r', 'MarkerSize', 10); hold on; 
%     else
%         plot(D,tan(psi),'.g', 'MarkerSize', 10); hold on; 
%     end
else
    dalpha = 0;
    dalpha2 = 0;
    comp = 0;
    comp2 = 0;
    params = 0;
    
    comp = x;
    comp2 = y;
    dalpha = theta;
end

% %% heuristics
% k_dang = 5;
% if  (A*x+B*y+C < 0) && (goawayflag == 0) && (~isAttrDomain)
%     d_comp = 0.1;
%     if (comp >= 0.8 + d_comp)
%         v = + 0.4;
%     elseif (comp <= 0.8 - d_comp)
%         v = - 0.35;
%     else
%         v = vlast;
%     end
%     
%     if (v > 0)
%         u = -k_dang*tan(dalpha); 
%     elseif params~=0
%         u = -params/Rmin; 
%     else
%         u = -sign(tau0 - thetas)/Rmin; 
%     end
% 
%     
% elseif (goawayflag == 1) && (~isAttrDomain)
%     if comp2 > 0 
%         v = - 0.3; 
%         u = k_dang*tan(dalpha2);
%     else 
%         v = + 0.3;
%         u = -k_dang*tan(dalpha2);
%     end   
% elseif (isAttrDomain)
% %% continue with spline following
%     %% Spline
% 
%     z1 = D;
%     z2 = sin(psi);
%     sigma = 2*lambda*z2+lambda*lambda*z1;
%     cospsi = cos(psi);
% 
%     u = K*cospsi/(K*z1+1) + (-sigma)/cospsi;
%     v = 0.6;
%     
% else
%     v = 0;
% %     u = 0;
%     error('NotAttrDomain');
% end
% 
% alpha = atan2(u*H,1);
% if alpha>thrhld
%     alpha=thrhld;
% elseif alpha<-thrhld
%     alpha=-thrhld;
% end    
%     
% u = tan(alpha)/H;
% 
% % u = ulast + 0.3*(u-ulast)*0.01;
% % v = vlast + 0.3*(v-vlast)*0.01;
% 
% ulast = u;
% vlast = v;

%% Auxiliary functions

function N = NormVec(A, varargin)
if nargin == 1
    % RotM = [0 -1; 1 0]; %Rotation of Vec A to -90 degrees
    RotM = [0 +1; -1 0]; %Rotation of Vec A to +90 degrees

else
    par =  varargin{1};
    if par == 1
        RotM = [0 +1; -1 0]; %Rotation of Vec A to +90 degrees
    elseif par == -1
        RotM = [0 -1; 1 0]; %Rotation of Vec A to -90 degrees
    else
        error("Normvec wrong parameter");
    end
end
    N = A'*RotM;
    N = N';
end

function [ANG2] = AngbwVec(R1,R2)
cos_ang = R1'*R2/(sqrt(R1'*R1)*sqrt(R2'*R2));

if cos_ang>1
    cos_ang=1;
elseif cos_ang<-1
    cos_ang=-1;
end

ANG = min(acos(cos_ang),pi-acos(cos_ang));
ANG2 = acos(cos_ang);
end


function ANG = AngSign(R1,R2) %% ----->>>> ERROR HERE ----- ERROR HERE <<<<-----
%signed angle [-pi, pi]
sin_ang = (R1(1)*R2(2)-R1(2)*R2(1))/(sqrt(R1'*R1)*sqrt(R2'*R2));
if sin_ang>1
    sin_ang=1;
elseif sin_ang<-1
    sin_ang=-1;
end

cos_ang = R1'*R2/(sqrt(R1'*R1)*sqrt(R2'*R2));   
if cos_ang>1
    cos_ang=1;
elseif cos_ang<-1
    cos_ang=-1;
end

if sin_ang == 0
    signang = 1;    
else
    signang = sign(sin_ang);
end

% ANG = acos(cos_ang)*sign(sin_ang);
ANG = acos(cos_ang)*signang;
end


function [Mt] = CrossPnt(R1,A1,R2,A2)
%Crossing point of two lines of A1 and A2
A = [A1(2), -A1(1); A2(2), -A2(1)];
b = [R1(1)*A1(2)-R1(2)*A1(1); R2(1)*A2(2)-R2(2)*A2(1)];
Mt = A\b;
end

function [Mn] = NorCrossPnt(R1,A1,R2,A2)
%Crossing point of two normal to A1 and A2
if AngbwVec(A1,A2)<pi/720
    Mn = [inf;inf];
    return
end
A = [A1'; A2'];
b = [R1'*A1; R2'*A2];
Mn = A\b;
end

function PlotLine(R1,R2)
line([R1(1) R2(1)], [R1(2), R2(2)],'Color','red','LineStyle','--');
end

function [eta, D,K,psi] = DKPsi(X,orient,calcEta,R,dR,ddR,phi,PHI,Xc)
    eta = 0;
if ( (isinf(Xc(1)) || isinf(Xc(2))) )
    UnityNormVec = NormVec(dR(0))/norm(NormVec(dR(0)));
    D = (X - R(0))'*UnityNormVec;
    K = 0;
    psi = AngSign(dR(0),orient);
%     tau = AngSign(dR(0),[1;0]);
    return
elseif norm(X - Xc)<1e-10 %% singular point => take D,K,tau from start of spline
    UnityNormVec = NormVec(dR(0))/norm(NormVec(dR(0)));
    D = (X - R(0))'*UnityNormVec;
    K = Cur(dR(0),ddR(0));
    psi = AngSign(dR(0),orient);
%     tau = AngSign(dR(0),[1;0]);
    return
end
    tx0 = phi/PHI;
    dtx = (X - R(tx0))'*NormVec(X-Xc)/((dR(tx0))'*NormVec(X-Xc));
    UnityNormVec = NormVec(dR(tx0+dtx))/norm(NormVec(dR(tx0+dtx)));

    D = (X - R(tx0+dtx))'*UnityNormVec;
    K = Cur(dR(tx0+dtx),ddR(tx0+dtx));
    psi = AngSign(dR(tx0+dtx),orient);
    eta = calcEta(tx0+dtx);
%     tau = AngSign(dR(tx0+dtx),[1;0]);
    
% hold on;
% S = R(tx0+dtx);
% plot(S(1),S(2), 'o');
% Xnplt = S+UnityNormVec;
% Xtauplt = S+dR(tx0+dtx)/norm(dR(tx0+dtx));
% plot(Xnplt(1),Xnplt(2), 'g^');
% plot(Xtauplt(1),Xtauplt(2), 'm<');
% hold off;
end

function K = Cur(dR,ddR)
K = (dR(1)*ddR(2)-dR(2)*ddR(1))/(dR'*dR)^(3/2);
end

function value = r(i,t)
value = 0;
if i >= 2 && i <= ((size(input,1)-2))
value = [transpose(input(i-1,:)),transpose(input(i,:)),transpose(input(i+1,:)),transpose(input(i+2,:))]*M*[1;t;t^2;t^3];
elseif i == 1
value = transpose(input(i,:))+(r(2,0)-transpose(input(i,:)))*t;
end
end

function value = dr(i,t)
value = 0;
if i >= 2 && i <= ((size(input,1)-2))
value = [transpose(input(i-1,:)),transpose(input(i,:)),transpose(input(i+1,:)),transpose(input(i+2,:))]*M*[0;1;2*t;3*t^2];
end    
end

function value = ddr(i,t)
value = 0;
if i >= 2 && i <= ((size(input,1)-2))
value = [transpose(input(i-1,:)),transpose(input(i,:)),transpose(input(i+1,:)),transpose(input(i+2,:))]*M*[0;0;2;6*t];
end    
end

function [dist] = distPLsign(X, R, dR) %%%%   ---->>>>> distance sign should be checked!! <<< ----
% Distance from point to line signed with according to NormVec(dR)
    UnityNormVec = NormVec(dR)/norm(NormVec(dR));
 
    dist = (X-R)'*UnityNormVec;
end

function [xc,yc,R] = BuildCircle(x,y,x0,y0,tau)
% AA = [(2*x-2*x0), (2*y-2*y0);
%       -cos(tau), -sin(tau) ];
if (-sin(tau)*(x-x0)+cos(tau)*(y-y0)) == 0
    error("BuildCircle error");
end

bb = [x^2+y^2-x0^2-y0^2; -cos(tau)*x0-sin(tau)*y0];

AA1 = [-sin(tau)/2 , -(y-y0);
      cos(tau)/2   ,  (x-x0)]/(-sin(tau)*(x-x0)+cos(tau)*(y-y0));
  
% xx = AA\bb;
xx = AA1*bb;

xc = xx(1);
yc = xx(2);
R = sqrt((x0-xc)^2+(y0-yc)^2);
end

function eta = calcEta(i,t)
eta = 0;
    if i >= 2 && i <= ((size(input,1)-2))
        for n = 2:i-1
            eta = eta + norm(input(n-1,:) - input(n,:));
        end
        eta = eta + t*norm(input(i-1,:) - input(i,:));
    end
end

end
